simulink subsystem "analogStates"  (R2022b)
settings: Solver=VariableStepAuto  StartTime=0.0  StopTime=10.0  RelTol=1e-3
settings Model: Creator=serga  LastModifiedBy=serga

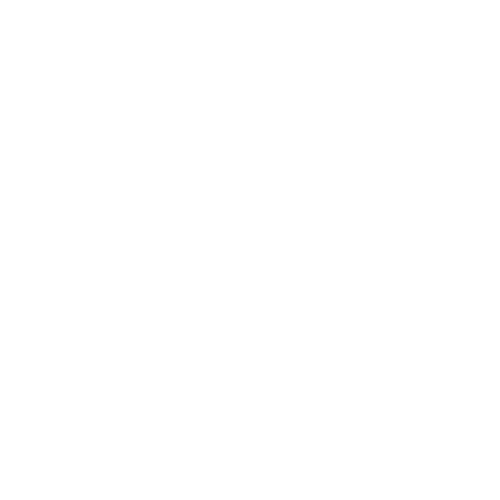
[thumbnail: Simulink's stored preview of the top-level diagram]
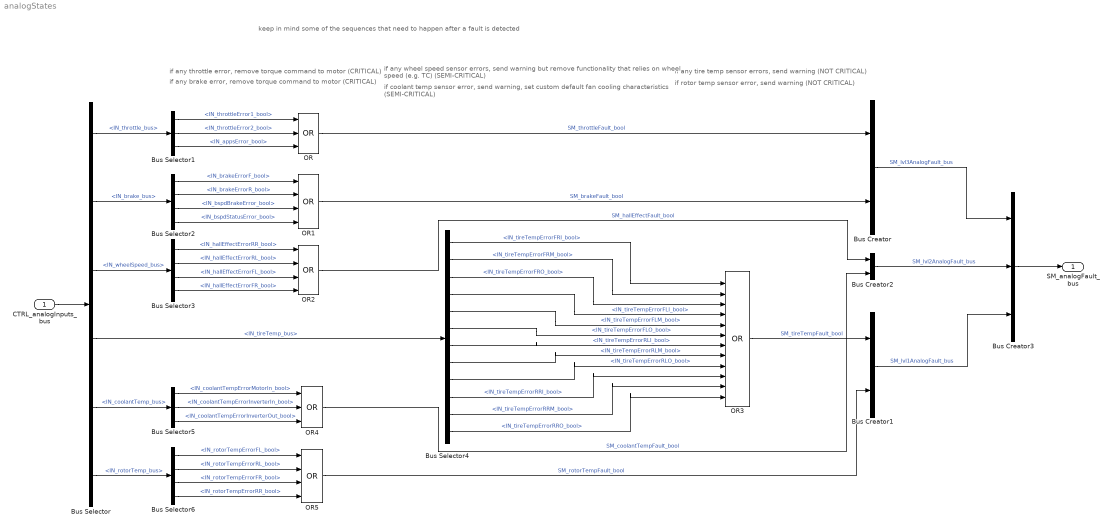
== system analogStates ==
  note: keep in mind some of the sequences that need to happen after a fault is detected
  note: if rotor temp sensor error, send warning (NOT CRITICAL)
  note: if coolant temp sensor error, send warning, set custom default fan cooling characteristics (SEMI-CRITICAL)
  note: if any tire temp sensor errors, send warning (NOT CRITICAL)
  note: if any wheel speed sensor errors, send warning but remove functionality that relies on wheel speed (e.g. TC) (SEMI-CRITICAL)
  note: if any brake error, remove torque command to motor (CRITICAL)
  note: if any throttle error, remove torque command to motor (CRITICAL)
  CTRL_analogInputs_bus : Inport
  Bus Creator : BusCreator  Inputs=2
  Bus Creator1 : BusCreator  Inputs=2
  Bus Creator2 : BusCreator  Inputs=2
  Bus Creator3 : BusCreator  Inputs=3
  Bus Selector : BusSelector  OutputSignals=IN_throttle_bus,IN_brake_bus,IN_wheelSpeed_bus,IN_tireTemp_bus,IN_coolantTemp_bus,IN_rotorTemp_bus
  Bus Selector1 : BusSelector  OutputSignals=IN_throttle1_bus.IN_throttleError1_bool,IN_throttle2_bus.IN_throttleError2_bool,IN_appsError_bool
  Bus Selector2 : BusSelector  OutputSignals=IN_brakeF_bus.IN_brakeErrorF_bool,IN_brakeR_bus.IN_brakeErrorR_bool,IN_bspdError_bus.IN_bspdBrakeError_bool,IN_bspdError_bus.IN_bspdStatusError_bool
  Bus Selector3 : BusSelector  OutputSignals=IN_wheelSpeedRR_bus.IN_hallEffectErrorRR_bool,IN_wheelSpeedRL_bus.IN_hallEffectErrorRL_bool,IN_wheelSpeedFL_bus.IN_hallEffectErrorFL_bool,IN_wheelSpeedFR_bus.IN_hallEffectErrorFR_bool
  Bus Selector4 : BusSelector  OutputSignals=IN_tireTempFR_bus.IN_tireTempFRI_bus.IN_tireTempErrorFRI_bool,IN_tireTempFR_bus.IN_tireTempFRM_bus.IN_tireTempErrorFRM_bool,IN_tireTempFR_bus.IN_tireTempFRO_bus.IN_tireTempErrorFRO_bool,IN_tireTempFL_bus.IN_tireTempFLI_bus.IN_tireTempErrorFLI_bool,IN_tireTempFL_bus.IN_tireTempFLM_bus.IN_tireTempErrorFLM_bool,IN_tireTempFL_bus.IN_tireTempFLO_bus.IN_tireTempErrorFLO_bool,IN_tireTempRL_bus.IN_tireTempRLI_bus.IN_tireTempErrorRLI_bool,IN_tireTempRL_bus.IN_tireTempRLM_bus.IN_tireTempErrorRLM_bool,IN_tireTempRL_bus.IN_tireTempRLO_bus.IN_tireTempErrorRLO_bool,IN_tireTempRR_bus.IN_tireTempRRI_bus.IN_tireTempErrorRRI_bool,IN_tireTempRR_bus.IN_tireTempRRM_bus.IN_tireTempErrorRRM_bool,IN_tireTempRR_bus.IN_tireTempRRO_bus.IN_tireTempErrorRRO_bool
  Bus Selector5 : BusSelector  OutputSignals=IN_coolantTempMotorIn_bus.IN_coolantTempErrorMotorIn_bool,IN_coolantTempInverterIn_bus.IN_coolantTempErrorInverterIn_bool,IN_coolantTempInverterOut_bus.IN_coolantTempErrorInverterOut_bool
  Bus Selector6 : BusSelector  OutputSignals=IN_rotorTempFL_bus.IN_rotorTempErrorFL_bool,IN_rotorTempRL_bus.IN_rotorTempErrorRL_bool,IN_rotorTempFR_bus.IN_rotorTempErrorFR_bool,IN_rotorTempRR_bus.IN_rotorTempErrorRR_bool
  OR : Logic  Operator=OR  Inputs=3  IconShape=distinctive  AllPortsSameDT=off  OutDataTypeStr=boolean
  OR1 : Logic  Operator=OR  Inputs=4  IconShape=distinctive  AllPortsSameDT=off  OutDataTypeStr=boolean
  OR2 : Logic  Operator=OR  Inputs=4  IconShape=distinctive  AllPortsSameDT=off  OutDataTypeStr=boolean
  OR3 : Logic  Operator=OR  Inputs=12  IconShape=distinctive  AllPortsSameDT=off  OutDataTypeStr=boolean
  OR4 : Logic  Operator=OR  Inputs=3  IconShape=distinctive  AllPortsSameDT=off  OutDataTypeStr=boolean
  OR5 : Logic  Operator=OR  Inputs=4  IconShape=distinctive  AllPortsSameDT=off  OutDataTypeStr=boolean
  SM_analogFault_bus : Outport
  wires:
  CTRL_analogInputs_bus/1 -> Bus Selector/1
  Bus Selector/1 -> Bus Selector1/1  "<IN_throttle_bus>"
  Bus Selector/2 -> Bus Selector2/1  "<IN_brake_bus>"
  Bus Selector/3 -> Bus Selector3/1  "<IN_wheelSpeed_bus>"
  Bus Selector/4 -> Bus Selector4/1  "<IN_tireTemp_bus>"
  Bus Selector/5 -> Bus Selector5/1  "<IN_coolantTemp_bus>"
  Bus Selector/6 -> Bus Selector6/1  "<IN_rotorTemp_bus>"
  Bus Selector1/1 -> OR/1  "<IN_throttleError1_bool>"
  Bus Selector1/2 -> OR/2  "<IN_throttleError2_bool>"
  Bus Selector1/3 -> OR/3  "<IN_appsError_bool>"
  Bus Selector2/1 -> OR1/1  "<IN_brakeErrorF_bool>"
  Bus Selector2/2 -> OR1/2  "<IN_brakeErrorR_bool>"
  Bus Selector2/3 -> OR1/3  "<IN_bspdBrakeError_bool>"
  Bus Selector2/4 -> OR1/4  "<IN_bspdStatusError_bool>"
  Bus Selector3/1 -> OR2/1  "<IN_hallEffectErrorRR_bool>"
  Bus Selector3/2 -> OR2/2  "<IN_hallEffectErrorRL_bool>"
  Bus Selector3/3 -> OR2/3  "<IN_hallEffectErrorFL_bool>"
  Bus Selector3/4 -> OR2/4  "<IN_hallEffectErrorFR_bool>"
  Bus Selector4/1 -> OR3/1  "<IN_tireTempErrorFRI_bool>"
  Bus Selector4/2 -> OR3/2  "<IN_tireTempErrorFRM_bool>"
  Bus Selector4/3 -> OR3/3  "<IN_tireTempErrorFRO_bool>"
  Bus Selector4/4 -> OR3/4  "<IN_tireTempErrorFLI_bool>"
  Bus Selector4/5 -> OR3/5  "<IN_tireTempErrorFLM_bool>"
  Bus Selector4/6 -> OR3/6  "<IN_tireTempErrorFLO_bool>"
  Bus Selector4/7 -> OR3/7  "<IN_tireTempErrorRLI_bool>"
  Bus Selector4/8 -> OR3/8  "<IN_tireTempErrorRLM_bool>"
  Bus Selector4/9 -> OR3/9  "<IN_tireTempErrorRLO_bool>"
  Bus Selector4/10 -> OR3/10  "<IN_tireTempErrorRRI_bool>"
  Bus Selector4/11 -> OR3/11  "<IN_tireTempErrorRRM_bool>"
  Bus Selector4/12 -> OR3/12  "<IN_tireTempErrorRRO_bool>"
  Bus Selector5/1 -> OR4/1  "<IN_coolantTempErrorMotorIn_bool>"
  Bus Selector5/2 -> OR4/2  "<IN_coolantTempErrorInverterIn_bool>"
  Bus Selector5/3 -> OR4/3  "<IN_coolantTempErrorInverterOut_bool>"
  Bus Selector6/1 -> OR5/1  "<IN_rotorTempErrorFL_bool>"
  Bus Selector6/2 -> OR5/2  "<IN_rotorTempErrorRL_bool>"
  Bus Selector6/3 -> OR5/3  "<IN_rotorTempErrorFR_bool>"
  Bus Selector6/4 -> OR5/4  "<IN_rotorTempErrorRR_bool>"
  Bus Creator/1 -> Bus Creator3/1  "SM_lvl3AnalogFault_bus"
  OR/1 -> Bus Creator/1  "SM_throttleFault_bool"
  OR1/1 -> Bus Creator/2  "SM_brakeFault_bool"
  OR3/1 -> Bus Creator1/1  "SM_tireTempFault_bool"
  OR5/1 -> Bus Creator1/2  "SM_rotorTempFault_bool"
  OR2/1 -> Bus Creator2/1  "SM_hallEffectFault_bool"
  OR4/1 -> Bus Creator2/2  "SM_coolantTempFault_bool"
  Bus Creator2/1 -> Bus Creator3/2  "SM_lvl2AnalogFault_bus"
  Bus Creator1/1 -> Bus Creator3/3  "SM_lvl1AnalogFault_bus"
  Bus Creator3/1 -> SM_analogFault_bus/1
